simulink model "model_00"  (R2014a)
settings: Solver=FixedStepDiscrete  StartTime=0.0  StopTime=SimLength  FixedStep=SampleTime  RelTol=1e-3
undefined symbols (not defined in the file): SimLength
libraries: simulink x2
settings Model: Creator=Maik  LastModifiedBy=georg

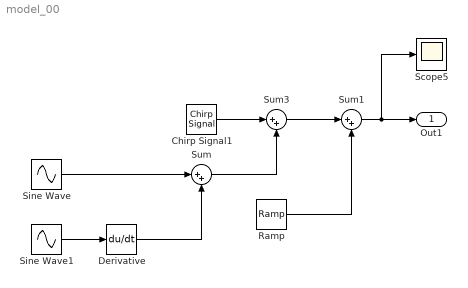
== system model_00 ==
  Chirp Signal1 : simulink/Sources/Chirp Signal  f1=0.1  T=SimLength  f2=1
  Derivative : Derivative
  Ramp : simulink/Sources/Ramp  slope=0.5  start=0  X0=0
  Scope5 : Scope
      settings: YMin=-1  YMax=1  SaveName=ScopeData5
  Sine Wave : Sin
  Sine Wave1 : Sin  Frequency=sqrt(3)
  Sum : Sum  Inputs=|++
  Sum1 : Sum  Inputs=|++
  Sum3 : Sum  Inputs=|++
  Out1 : Outport
  wires:
  Sine Wave1/1 -> Derivative/1
  Sine Wave/1 -> Sum/1
  Derivative/1 -> Sum/2
  Sum/1 -> Sum3/2
  Chirp Signal1/1 -> Sum3/1
  Ramp/1 -> Sum1/2
  Sum3/1 -> Sum1/1
  Sum1/1 -> Scope5/1, Out1/1
